simulink model "model"  (R2021a)
settings: Solver=ode4  StartTime=0.0  StopTime=simtime  FixedStep=0.001  RelTol=1e-3
values from neighbouring files (symbols this model uses):
  A = [0 1 0 0 0 ... (first row only)    [assignment_3.m]
  B = [B1 B2]    [assignment_3.m]
  C = eye(5)    [assignment_3.m]
  Cf = 2*60000    (= 120000)    [assignment_3.m]
  Cr = 2*57000    (= 114000)    [assignment_3.m]
  D = zeros(5,2)    [assignment_3.m]
  delay = 1    [assignment_3.m]
  Kff = ((mv*Vx^2)/l)*((lr/Cf)-(lf/Cr)+(lf*K_g(3)/Cr))+l-(lr*K_g(3))    [assignment_3.m]
  l = lr+lf    (= 2.8)    [assignment_3.m]
  lf = 1.3    [assignment_3.m]
  lr = 1.5    [assignment_3.m]
  mv = 1575    [assignment_3.m]
  ref = 1    [assignment_3.m]
  Vx = 80/3.6    (= 22.2222222222)    [assignment_3.m]
  x0 = zeros(4,1)    [assignment_3.m]
undefined symbols (not defined in the file or in its folder): K
libraries: simulink_extras x2, simulink x1
settings Model: Creator=Giacomo  LastModifiedBy=Utente
settings DataIOCC: ReturnWorkspaceOutputs=off
settings DebuggingCC: UnconnectedInputMsg=none  UnconnectedOutputMsg=none  UnconnectedLineMsg=none
settings RTWCC: DLArmComputeVersion=20.02.1

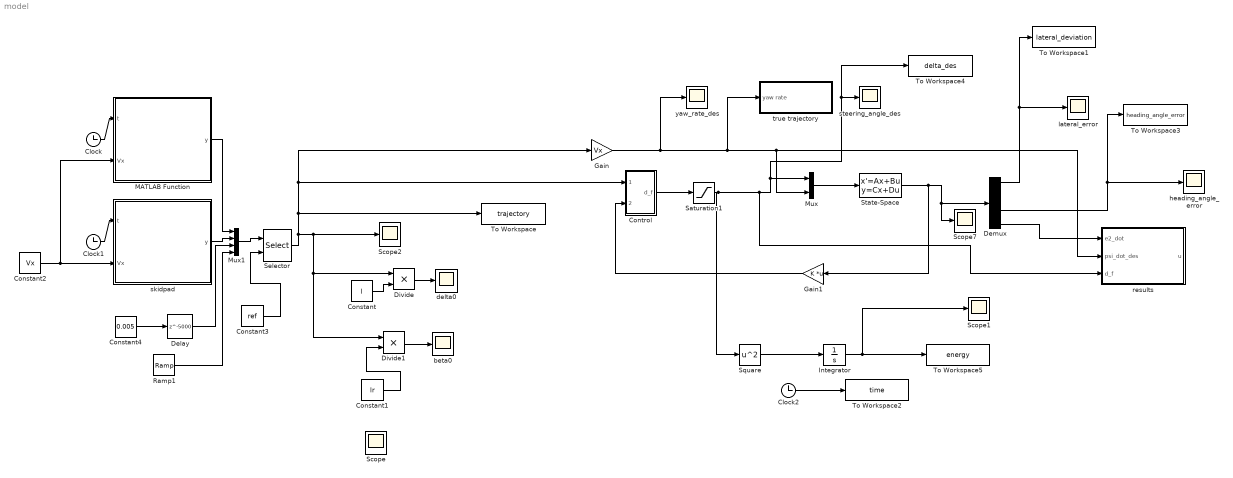
== system model ==
  Clock : Clock
  Clock1 : Clock
  Clock2 : Clock
  Constant : Constant  Value=l
  Constant1 : Constant  Value=lr
  Constant2 : Constant  Value=Vx
  Constant3 : Constant  Value=ref
  Constant4 : Constant  Value=0.005
  Control : Subsystem
  Delay : Delay  DelayLength=5000
  Demux : Demux
  Divide : Product
  Divide1 : Product
  Gain : Gain  Gain=Vx
  Gain1 : Gain  Gain=K  Multiplication=Matrix(K*u) (u vector)
  Integrator : Integrator
  MATLAB Function : MATLAB Function  TreatAsAtomicUnit=on
  Mux : Mux  Inputs=2
  Mux1 : Mux
  Ramp1 : simulink/Sources/Ramp  slope=0.0012  start=5  InitialOutput=0
  Saturation1 : Saturate  UpperLimit=25*pi/180  LowerLimit=-25*pi/180
  Scope{,1..2,7} (4 alike) : Scope
  Selector : Selector  InputPortWidth=4  IndexOptions=Index vector (port)  Indices=1  OutputSizes=1
  Square : Math  Operator=square  SaturateOnIntegerOverflow=on
  State-Space : StateSpace  A=A  B=B  C=C  D=D  InitialCondition=x0
  To Workspace : ToWorkspace  VariableName=trajectory  SampleTime=-1
  To Workspace1 : ToWorkspace  VariableName=lateral_deviation  SampleTime=-1
  To Workspace2 : ToWorkspace  VariableName=time  SampleTime=-1
  To Workspace3 : ToWorkspace  VariableName=heading_angle_error  SampleTime=-1
  To Workspace4 : ToWorkspace  VariableName=delta_des  SampleTime=-1
  To Workspace5 : ToWorkspace  VariableName=energy  SampleTime=-1
  beta0 : Scope
  delta0 : Scope
  heading_angle_error : Scope
  lateral_error : Scope
  results : Subsystem
  skidpad : MATLAB Function  TreatAsAtomicUnit=on
  steering_angle_des : Scope
  true trajectory : Subsystem
  yaw_rate_des : Scope
  wires:
  Clock/1 -> MATLAB Function/1(t)
  Gain/1 -> true trajectory/1(yaw rate), results/2(psi_dot_des), Mux/2, yaw_rate_des/1
  Constant/1 -> Divide/2
  Divide/1 -> delta0/1
  Divide1/1 -> beta0/1
  Constant1/1 -> Divide1/2
  Control/1(d_f) -> Saturation1/1
  Clock1/1 -> skidpad/1(t)
  Constant2/1 -> MATLAB Function/2(Vx), skidpad/2(Vx)
  Mux1/1 -> Selector/1
  MATLAB Function/1(y) -> Mux1/1
  skidpad/1(y) -> Mux1/2
  Ramp1/1 -> Mux1/4
  Constant3/1 -> Selector/2
  Gain1/1 -> Control/2(In2)
  State-Space/1 -> Scope7/1, Demux/1, Gain1/1
  Mux/1 -> State-Space/1
  Demux/1 -> To Workspace1/1, lateral_error/1
  Demux/3 -> To Workspace3/1, heading_angle_error/1
  Demux/4 -> results/1(e2_dot)
  Selector/1 -> Gain/1, Control/1(In1), To Workspace/1, Divide/1, Divide1/1, Scope2/1
  Clock2/1 -> To Workspace2/1
  Constant4/1 -> Delay/1
  Delay/1 -> Mux1/3
  Integrator/1 -> Scope1/1, To Workspace5/1
  Saturation1/1 -> Square/1, results/3(d_f), Mux/1, To Workspace4/1, steering_angle_des/1
  Square/1 -> Integrator/1

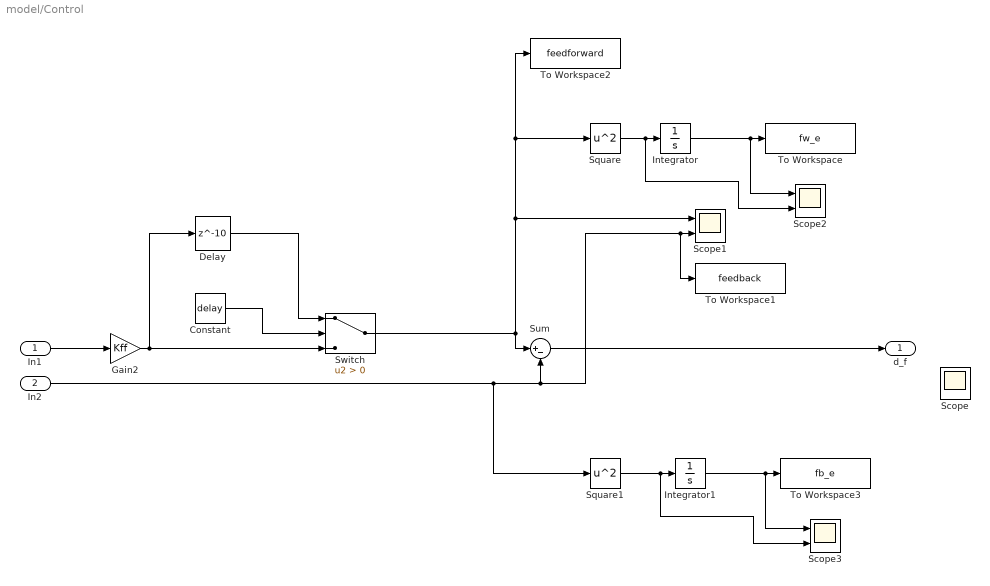
== system model/Control ==
  In1 : Inport
  In2 : Inport  Port=2
  Constant : Constant  Value=delay
  Delay : Delay  DelayLength=10
  Gain2 : Gain  Gain=Kff
  Integrator : Integrator
  Integrator1 : Integrator
  Scope : Scope
  Scope1 : Scope  NumInputPorts=2
  Scope2 : Scope  NumInputPorts=2
  Scope3 : Scope  NumInputPorts=2
  Square : Math  Operator=square  SaturateOnIntegerOverflow=on
  Square1 : Math  Operator=square  SaturateOnIntegerOverflow=on
  Sum : Sum  Inputs=|+-
  Switch : Switch  Criteria=u2 > Threshold
  To Workspace : ToWorkspace  VariableName=fw_e  SampleTime=-1
  To Workspace1 : ToWorkspace  VariableName=feedback  SampleTime=-1
  To Workspace2 : ToWorkspace  VariableName=feedforward  SampleTime=-1
  To Workspace3 : ToWorkspace  VariableName=fb_e  SampleTime=-1
  d_f : Outport
  wires:
  In1/1 -> Gain2/1
  Sum/1 -> d_f/1
  Gain2/1 -> Delay/1, Switch/3
  Delay/1 -> Switch/1
  Constant/1 -> Switch/2
  Switch/1 -> Sum/1, Square/1, To Workspace2/1, Scope1/1
  Integrator/1 -> Scope2/1, To Workspace/1
  Integrator1/1 -> Scope3/1, To Workspace3/1
  In2/1 -> Square1/1, Sum/2, To Workspace1/1, Scope1/2
  Square1/1 -> Scope3/2, Integrator1/1
  Square/1 -> Scope2/2, Integrator/1

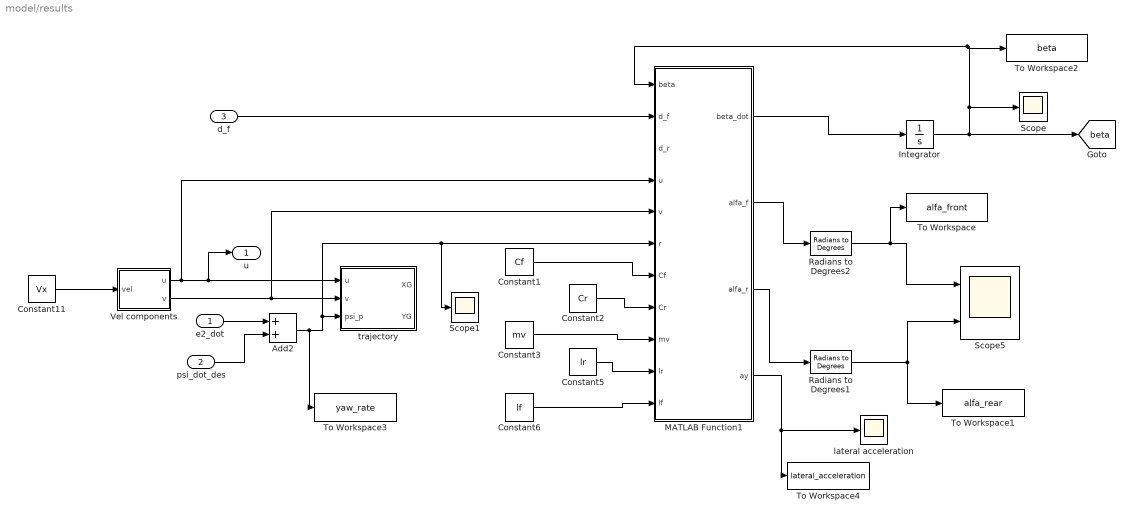
== system model/results ==
  e2_dot : Inport
  psi_dot_des : Inport  Port=2
  d_f : Inport  Port=3
  Add2 : Sum
  Constant1 : Constant  Value=Cf
  Constant11 : Constant  Value=Vx
  Constant2 : Constant  Value=Cr
  Constant3 : Constant  Value=mv
  Constant5 : Constant  Value=lr
  Constant6 : Constant  Value=lf
  Integrator : Integrator
  MATLAB Function1 : MATLAB Function  TreatAsAtomicUnit=on
  Radians to Degrees1 : simulink_extras/Transformations/Radians to Degrees
  Radians to Degrees2 : simulink_extras/Transformations/Radians to Degrees
  Scope : Scope
  Scope1 : Scope
  Scope5 : Scope  NumInputPorts=2
  To Workspace : ToWorkspace  VariableName=alfa_front  SampleTime=-1
  To Workspace1 : ToWorkspace  VariableName=alfa_rear  SampleTime=-1
  To Workspace2 : ToWorkspace  VariableName=beta  SampleTime=-1
  To Workspace3 : ToWorkspace  VariableName=yaw_rate  SampleTime=-1
  To Workspace4 : ToWorkspace  VariableName=lateral_acceleration  SampleTime=-1
  Vel components : Subsystem
  lateral acceleration : Scope
  trajectory : Subsystem
  u : Outport
  tag scope: beta=global
  wires:
  Integrator/1 -> [beta], To Workspace2/1, MATLAB Function1/1(beta), Scope/1
  psi_dot_des/1 -> Add2/2
  e2_dot/1 -> Add2/1
  d_f/1 -> MATLAB Function1/2(d_f)
  Constant1/1 -> MATLAB Function1/7(Cf)
  Constant2/1 -> MATLAB Function1/8(Cr)
  Radians to Degrees2/1 -> To Workspace/1, Scope5/1
  MATLAB Function1/3(alfa_r) -> Radians to Degrees1/1
  Radians to Degrees1/1 -> To Workspace1/1, Scope5/2
  Constant3/1 -> MATLAB Function1/9(mv)
  Constant6/1 -> MATLAB Function1/11(lf)
  MATLAB Function1/2(alfa_f) -> Radians to Degrees2/1
  Vel components/2(v) -> MATLAB Function1/5(v), trajectory/2(v)
  Constant5/1 -> MATLAB Function1/10(lr)
  Constant11/1 -> Vel components/1(vel)
  Add2/1 -> To Workspace3/1, Scope1/1, MATLAB Function1/6(r), trajectory/3(psi_p)
  Vel components/1(u) -> u/1, trajectory/1(u), MATLAB Function1/4(u)
  MATLAB Function1/1(beta_dot) -> Integrator/1
  MATLAB Function1/4(ay) -> To Workspace4/1, lateral acceleration/1

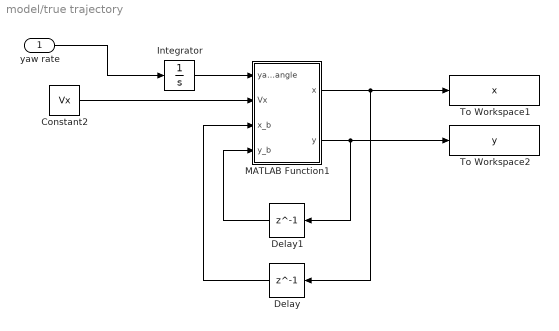
== system model/true trajectory ==
  yaw rate : Inport
  Constant2 : Constant  Value=Vx
  Delay : Delay  DelayLength=1
  Delay1 : Delay  DelayLength=1
  Integrator : Integrator
  MATLAB Function1 : MATLAB Function  TreatAsAtomicUnit=on
  To Workspace1 : ToWorkspace  VariableName=x  SampleTime=-1
  To Workspace2 : ToWorkspace  VariableName=y  SampleTime=-1
  wires:
  MATLAB Function1/2(y) -> To Workspace2/1, Delay1/1
  MATLAB Function1/1(x) -> Delay/1, To Workspace1/1
  Constant2/1 -> MATLAB Function1/2(Vx)
  Delay/1 -> MATLAB Function1/3(x_b)
  Integrator/1 -> MATLAB Function1/1(yaw_angle)
  Delay1/1 -> MATLAB Function1/4(y_b)
  yaw rate/1 -> Integrator/1

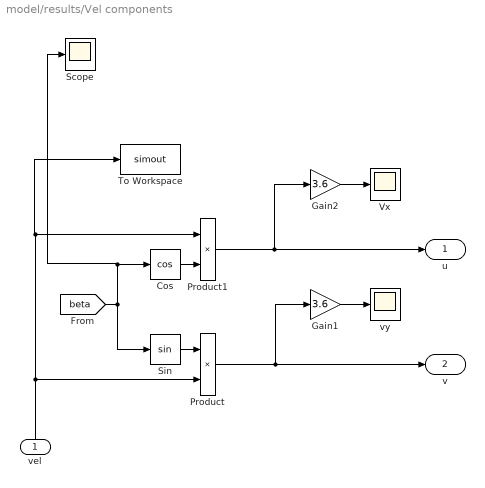
== system model/results/Vel components ==
  vel : Inport
  Cos : Trigonometry  Operator=cos
  Gain1 : Gain  Gain=3.6
  Gain2 : Gain  Gain=3.6
  Product : Product
  Product1 : Product
  Scope : Scope
  Sin : Trigonometry
  To Workspace : ToWorkspace  VariableName=simout  SaveFormat=Timeseries  SampleTime=-1
  Vx : Scope
  vy : Scope
  u : Outport  VectorParamsAs1DForOutWhenUnconnected=off
  v : Outport  Port=2  VectorParamsAs1DForOutWhenUnconnected=off
  wires:
  Product/1 -> Gain1/1, v/1
  vel/1 -> Product/2, Product1/1, To Workspace/1
  Gain1/1 -> vy/1
  Gain2/1 -> Vx/1
  Cos/1 -> Product1/2
  Product1/1 -> Gain2/1, u/1
  [beta] -> Sin/1, Scope/1, Cos/1
  Sin/1 -> Product/1

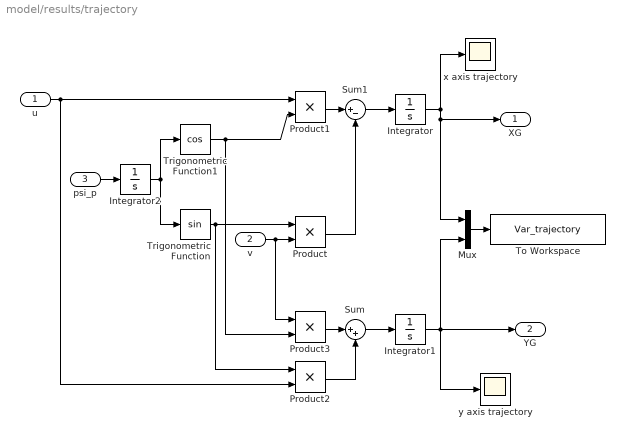
== system model/results/trajectory ==
  u : Inport
  v : Inport  Port=2
  psi_p : Inport  Port=3
  Integrator : Integrator
  Integrator1 : Integrator
  Integrator2 : Integrator
  Mux : Mux  Inputs=2
  Product{,1..3} (4 alike) : Product  InputSameDT=on  SaturateOnIntegerOverflow=on  OutDataTypeStr=Inherit: Same as first input
  Sum : Sum  Inputs=|++  InputSameDT=on  SaturateOnIntegerOverflow=on  OutDataTypeStr=Inherit: Same as first input
  Sum1 : Sum  Inputs=|+-  InputSameDT=on  SaturateOnIntegerOverflow=on  OutDataTypeStr=Inherit: Same as first input
  To Workspace : ToWorkspace  VariableName=Var_trajectory  SampleTime=-1
      settings: Save2DSignal=2-D array (concatenate along first dimension)
      settings: InitFcn=|
      | ParentName = get_param(gcb,'Parent');
      | cont = max(find(ParentName=='/'));
      | set_param(gcb,'VariableName',strcat('Var_',ParentName(cont+1:length(ParentName))));
      | clear ParentName cont
  Trigonometric Function : Trigonometry
  Trigonometric Function1 : Trigonometry  Operator=cos
  x axis trajectory : Scope
  y axis trajectory : Scope
  XG : Outport  VectorParamsAs1DForOutWhenUnconnected=off
  YG : Outport  Port=2  VectorParamsAs1DForOutWhenUnconnected=off
  wires:
  psi_p/1 -> Integrator2/1
  Product1/1 -> Sum1/1
  Product/1 -> Sum1/2
  Sum1/1 -> Integrator/1
  Trigonometric Function/1 -> Product/1, Product2/1
  u/1 -> Product2/2, Product1/1
  v/1 -> Product/2, Product3/1
  Trigonometric Function1/1 -> Product1/2, Product3/2
  Product3/1 -> Sum/1
  Product2/1 -> Sum/2
  Sum/1 -> Integrator1/1
  Integrator/1 -> XG/1, Mux/1, x axis trajectory/1
  Integrator1/1 -> YG/1, y axis trajectory/1, Mux/2
  Mux/1 -> To Workspace/1
  Integrator2/1 -> Trigonometric Function/1, Trigonometric Function1/1

== matlab function model/results/MATLAB Function1 ==
  data: beta input; d_f input; d_r input; u input; v input; r input; beta_dot output; alfa_f output; alfa_r output; Cf input; Cr input; mv input; lr input; lf input; ay output
function [beta_dot, alfa_f, alfa_r, ay] = fcn(beta,d_f,d_r,u,v,r,Cf,Cr,mv,lr,lf)
l = lr+lf; % total wheelbase

beta_dot = (-Cf - Cr)/(mv*u)*beta + (-Cf*lf + Cr*lr - mv*u^2)/(mv*u^2)*r + (Cf*d_f - Cr*d_r)/(mv*u);
alfa_f = -beta - (lf*r)/u + d_f;
alfa_r = - beta + (lr*r)/u + d_r;
%ay = -(Cf+Cr)/(mv*u)*v+(Cr*lr-Cf*lf-mv*u^2)/(mv*u)*r+Cf*d_f/mv;
ay = u*r;

== matlab function model/MATLAB Function ==
  data: t input; y output; Vx input
function y = fcn(t, Vx)
y = 0;
low = 0.002;

coeff=(80/3.6)/Vx;
t1=27*coeff;
if t <= t1
    y = 0;
end
if t >= t1
    y=(t-t1)*low/-(10*coeff);
end
t2=t1+(10*coeff);
if t >= t2
    y = -low;
end
t3=t2+(27*coeff);
if t >= t3
    y= (t-t3-(10*coeff))*low/(10*coeff);
end
t4=t3+(10*coeff);
if t >= t4
    y = 0;
end
t5=t4+(56*coeff);
if t >= t5
    y = (t5-t)*low/-(10*coeff);
end
t6=t5+(10*coeff);
if t >= t6
    y = low;
end
t7=t6+(30*coeff);
t8=t7+(10*coeff);
if t >= t7
    y = (t-t8)*low/-(10*coeff);
end
if t >= t8
    y = 0;
end

== matlab function model/true trajectory/MATLAB Function1 ==
  data: x output; yaw_angle input; Vx input; y output; x_b input; y_b input
function [x,y] = fcn(yaw_angle,Vx,x_b,y_b)
dt=0.001;

x=x_b+Vx*cos(yaw_angle)*dt;
y=y_b+Vx*sin(yaw_angle)*dt;

== matlab function model/skidpad ==
  data: t input; y output; Vx input
function y = fcn(t, Vx)
y = 0;
c=1000;
circ=(80/3.6)*60;
r=circ/(2*pi*2); %il secondo 2 è perché deve fare due giri
kl=1/r;

t1=((80/3.6)*10)/Vx;
if t <= t1
    y = 0;
end
t2=circ/Vx;
if t >= t1
    y = -kl;
end
if t >= t1+t2
    y = kl;
end
if t >= t1+2*t2
    y=0;
end
